simulink model "GreenCraneV1_mrhAdjust"  (R2025b)
settings: Solver=VariableStepAuto  StartTime=0.0  StopTime=40  RelTol=1e-3
model workspace (MATLAB code in the model file):
  | clear;
  | %% Hydraulics
  | 
  | %Liquid
  | rho = 875;
  | beta = 1000; %MPa
  | 
  | %Pump
  | pP = 6e6; %60 bar in pa
  | 
  | %Directional control valve
  | dp0 = 7e5; %Nominal pressure drop, Pa (stod 70e5)
  | Q0 = 10/6e4; %Nominal flow, m^3/s
  | Cd = 0.75; %Discharge coefficient
  | AdMax_SI = Q0/(Cd*(2/rho*dp0)^0.5); %Discharge area m^2
  | AdMax = AdMax_SI*1e6;
  | 
  | %cylinders (dummy)
  | d = 80; %mm
  | dr = 50; %mm
  | A = pi*d^2/4;
  | Ar = pi*dr^2/4;
  | Aa = A - Ar;
  | L0 = 1600; %mm
  | 
  | %Weight (bruker ikke lenger?)
  | m = 75*4 + 20 + 90; %kg
  | g = 9.81; %m/s^2
  | MG = m*g; %Force from weight
  | %inital postition
  | x_Init = 200; %mm
  | 
  | %% Geometric properties
  | 
  | % Cylinder Translation
  | Cx = 427; %mm translation from global coordinate
  | Cz = -1057; %mm translation
  | 
  | % Crane arm
  | theta_Init = 73.04- 90; %deg når kran er nede
  | thetaDot_Init = 0;
  | L1 = 3680; %mm length of beam
  | B1 = 100; %mm width of beam
  | H1 = 150; %mm height
  | t1 = 6; %mm thickness
  | revBasePinDia = 60; %mm of the pin in the main hinge
  | revBasePinLength = 185.5; %mm of the pin in the main hinge
  | 
  | %Cylinder
  | rEar = 35; %mm radius of the bearing ear
  | tEar = 30; %mm thickness of ear
  | earToCylTop = 52.45; %mm center of ear to top of cylinder in bottom pos
  | earToCylBot = 40.62; %mm center of ear to bottom cylinder in bottom pos
  | cylDia = 75; %mm Diameter of cylinger housing
  | cylLength = 682; %mm length of housing
  | rodLength = 565.26; %mm length of rod
  | rodDia = 35; %mm rod diameter
  | rodToCyl = 132; %mm Length in bottom pos from bottom of cylinder to bottom of rod without rod plate
  | revCylPinDia = 25; %mm diameter of the pin that the bearing of the top and bottom of cylinder revolves around
  | revCylPinLength = 84; %mm length of the pin
  | rPiston = 65/2; %mm radius of piston
  | tPiston = 40; %mm thickness of piston
  | 
  | %Ear top
  | abx = 564.99; %mm; in the bottom pos
  | aby = 133; %mm in the bottom pos
  | 
  | % PayLoad
  | L2 = 210; %mm of the whole weight block
  | B2 = 700; %mm
  | H2 = 300; %mm
  | dY_PL_Beam = 75; %mm center of beam to center of payload
  | 
  | %% Mass properties (mass and center of mass)
  | beam_mass = 410.675; %kg mass of payload and beam
  | beam_COM = [3043.56 63.40 0]; %mm
  | 
  | 
  | %% Inertia properties (Moments of inertia and products of inertia)
  | beam_MOI = [0.017432114  0.421942031  0.410722495];   % kg·m^2 Mulig feil rekkefølge
  | beam_POI = [0.011754324  -2.50964e-6  -5.072e-8];  % kg·m^2
  | %tro disse er i feil rekkefølge siden simscape bruker et annet aksesystem
undefined symbols (not defined in the file): X, Y, Z
libraries: sm_lib x37, fl_lib x16, nesl_utility x10, SimscapeFluids_lib x3
(part 2 of 2)

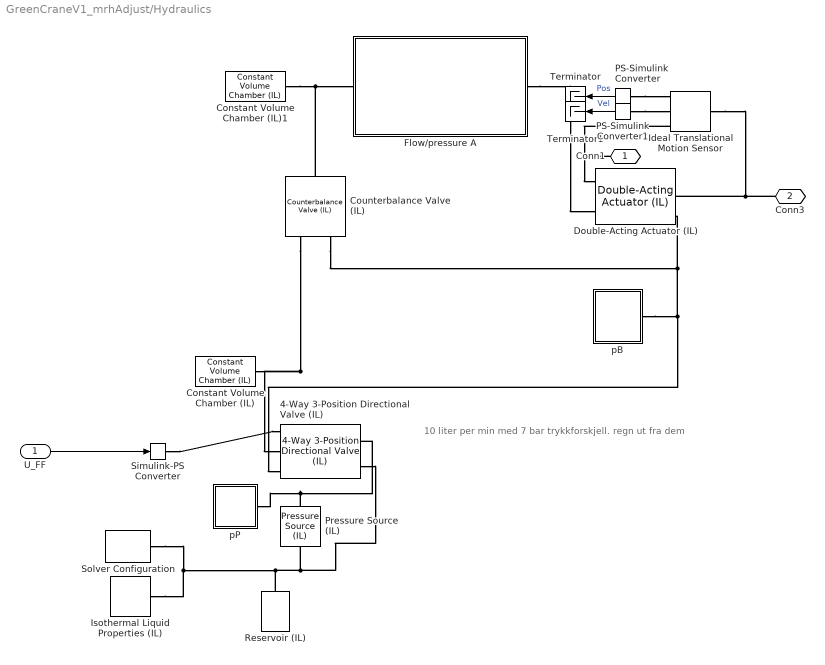
== system GreenCraneV1_mrhAdjust/Hydraulics ==
  note: 10 liter per min med 7 bar trykkforskjell. regn ut fra dem
  U_FF : Inport
  4-Way 3-Position Directional Valve (IL) : SimscapeFluids_lib/Isothermal Liquid/Valves & Orifices/Directional Control Valves/4-Way 3-Position Directional Valve (IL)  open_orifices_pos=fluids.isothermal_liquid.valves_orifices.directional_control_valves.enum.directional_valve_open_orifices_pos_neg.PA_BT  open_orifices_neu=fluids.isothermal_liquid.valves_orifices.directional_control_valves.enum.directional_valve_open_orifices_neutral.all_closed  open_orifices_neg=fluids.isothermal_liquid.valves_orifices.directional_control_valves.enum.directional_valve_open_orifices_pos_neg.PB_AT  neutral_assert_action=simscape.enum.assert.action.warn  area_spec=fluids.isothermal_liquid.valves_orifices.directional_control_valves.enum.directional_valve_area_spec.identical  valve_spec=fluids.isothermal_liquid.valves_orifices.directional_control_valves.enum.directional_valve_spec.linear  del_S_max=1 m  area_max=AdMax mm^2  del_S_TLU=[0, .00125, .0025, .00375, .005] m  valve_area_TLU=[1e-10, 1e-05, 4e-05, 6e-05, .0001] m^2  del_S_vol_flow_TLU=[0, .00125, .0025, .00375, .005] m  p_diff_TLU=[-.1, .3, .5, .7] MPa  vol_flow_TLU=[-1e-08, 2.2e-08, 2.8e-08, 3.4e-08; -9e-06, .00015, .0002, .00024; -.00036, .00063, .00081, .00096; -.00054, .00094, .0012, .0014; -.00091, .0016, .002, .0024] m^3/s  p_diff_TLU_const=[-.1, .3, .5, .7] MPa  vol_flow_TLU_const=[-.0009, .0016, .002, .0024] m^3/s  area_const=1e-4 m^2  area_leak=1e-10 m^2  area=inf m^2  Cd=Cd  Re_c=150  smoothing_factor=0.01  pressure_recovery=false  S_max_PA=1 m  del_S_max_PA=0.005 m  area_max_PA=1e-4 m^2  del_S_TLU_PA=[0, .00125, .0025, .00375, .005] m  valve_area_TLU_PA=[1e-10, 1e-05, 4e-05, 6e-05, .0001] m^2  del_S_vol_flow_TLU_PA=[0, .00125, .0025, .00375, .005] m  p_diff_TLU_PA=[-.1, .3, .5, .7] MPa  vol_flow_TLU_PA=[-1e-08, 2.2e-08, 2.8e-08, 3.4e-08; -9e-06, .00015, .0002, .00024; -.00036, .00063, .00081, .00096; -.00054, .00094, .0012, .0014; -.00091, .0016, .002, .0024] m^3/s  area_const_PA=1e-4 m^2  p_diff_TLU_const_PA=[-.1, .3, .5, .7] MPa  vol_flow_TLU_const_PA=[-.0009, .0016, .002, .0024] m^3/s  S_max_PB=-1 m  del_S_max_PB=0.005 m  area_max_PB=1e-4 m^2  del_S_TLU_PB=[0, .00125, .0025, .00375, .005] m  valve_area_TLU_PB=[1e-10, 1e-05, 4e-05, 6e-05, .0001] m^2  del_S_vol_flow_TLU_PB=[0, .00125, .0025, .00375, .005] m  p_diff_TLU_PB=[-.1, .3, .5, .7] MPa  vol_flow_TLU_PB=[-1e-08, 2.2e-08, 2.8e-08, 3.4e-08; -9e-06, .00015, .0002, .00024; -.00036, .00063, .00081, .00096; -.00054, .00094, .0012, .0014; -.00091, .0016, .002, .0024] m^3/s  area_const_PB=1e-4 m^2  p_diff_TLU_const_PB=[-.1, .3, .5, .7] MPa  vol_flow_TLU_const_PB=[-.0009, .0016, .002, .0024] m^3/s  S_max_AB=7.5e-3 m  del_S_max_AB=0.005 m  area_max_AB=1e-4 m^2  del_S_TLU_AB=[0, .00125, .0025, .00375, .005] m  valve_area_TLU_AB=[1e-10, 1e-05, 4e-05, 6e-05, .0001] m^2  del_S_vol_flow_TLU_AB=[0, .00125, .0025, .00375, .005] m  p_diff_TLU_AB=[-.1, .3, .5, .7] MPa  vol_flow_TLU_AB=[-1e-08, 2.2e-08, 2.8e-08, 3.4e-08; -9e-06, .00015, .0002, .00024; -.00036, .00063, .00081, .00096; -.00054, .00094, .0012, .0014; -.00091, .0016, .002, .0024] m^3/s  area_const_AB=1e-4 m^2  p_diff_TLU_const_AB=[-.1, .3, .5, .7] MPa  vol_flow_TLU_const_AB=[-.0009, .0016, .002, .0024] m^3/s  S_max_AT=-1 m  del_S_max_AT=0.005 m  area_max_AT=1e-4 m^2  del_S_TLU_AT=[0, .00125, .0025, .00375, .005] m  valve_area_TLU_AT=[1e-10, 1e-05, 4e-05, 6e-05, .0001] m^2  del_S_vol_flow_TLU_AT=[0, .00125, .0025, .00375, .005] m  p_diff_TLU_AT=[-.1, .3, .5, .7] MPa  vol_flow_TLU_AT=[-1e-08, 2.2e-08, 2.8e-08, 3.4e-08; -9e-06, .00015, .0002, .00024; -.00036, .00063, .00081, .00096; -.00054, .00094, .0012, .0014; -.00091, .0016, .002, .0024] m^3/s  area_const_AT=1e-4 m^2  p_diff_TLU_const_AT=[-.1, .3, .5, .7] MPa  vol_flow_TLU_const_AT=[-.0009, .0016, .002, .0024] m^3/s  S_max_BT=1 m  del_S_max_BT=0.005 m  area_max_BT=1e-4 m^2  del_S_TLU_BT=[0, .00125, .0025, .00375, .005] m  valve_area_TLU_BT=[1e-10, 1e-05, 4e-05, 6e-05, .0001] m^2  del_S_vol_flow_TLU_BT=[0, .00125, .0025, .00375, .005] m  p_diff_TLU_BT=[-.1, .3, .5, .7] MPa  vol_flow_TLU_BT=[-1e-08, 2.2e-08, 2.8e-08, 3.4e-08; -9e-06, .00015, .0002, .00024; -.00036, .00063, .00081, .00096; -.00054, .00094, .0012, .0014; -.00091, .0016, .002, .0024] m^3/s  area_const_BT=1e-4 m^2  p_diff_TLU_const_BT=[-.1, .3, .5, .7] MPa  vol_flow_TLU_const_BT=[-.0009, .0016, .002, .0024] m^3/s  S_max_PT=0 m  del_S_max_PT=0.005 m  area_max_PT=1e-4 m^2  del_S_TLU_PT=[0, .00125, .0025, .00375, .005] m  valve_area_TLU_PT=[1e-10, 1e-05, 4e-05, 6e-05, .0001] m^2  del_S_vol_flow_TLU_PT=[0, .00125, .0025, .00375, .005] m  p_diff_TLU_PT=[-.1, .3, .5, .7] MPa  vol_flow_TLU_PT=[-1e-08, 2.2e-08, 2.8e-08, 3.4e-08; -9e-06, .00015, .0002, .00024; -.00036, .00063, .00081, .00096; -.00054, .00094, .0012, .0014; -.00091, .0016, .002, .0024] m^3/s
      settings: InternalSimscapePortConfiguration="{\"Bottom\":[{\"id\":\"P\",\"label\":\"P\",\"type\":\"foundation.isothermal_liquid.isothermal_liquid\"},{\"id\":\"T\",\"label\":\"T\",\"type\":\"foundation.isothermal_liquid.isothermal_liquid\"}],\"Left\":[{\"id\":\"S\",\"label\":\"S\",\"type\":\"input\"}],\"Right\":[],\"Top\":[{\"id\":\"A\",\"label\":\"A\",\"type\":\"foundation.isothermal_liquid.isothermal_liquid\"},{\"id\":\"B\",\"label\":\"B\",\"type\":\"foundation.isothermal_liquid.isothermal_liquid\"}]}"
  Constant Volume Chamber (IL) : fl_lib/Isothermal Liquid/Elements/Constant Volume Chamber (IL)  volume=1 l  p_I_specify=on  p_I_priority=High  p_I=pP Pa  p_I_nominal_specify=off  p_I_nominal_value=1  p_I_nominal_unit=MPa
      settings: InternalSimscapePortConfiguration="{\"Bottom\":[],\"Left\":[{\"id\":\"A\",\"label\":\"A\",\"type\":\"foundation.isothermal_liquid.isothermal_liquid\"}],\"Right\":[],\"Top\":[]}"
  Constant Volume Chamber (IL)1 : fl_lib/Isothermal Liquid/Elements/Constant Volume Chamber (IL)  volume=1 l  p_I_specify=on  p_I_priority=High  p_I=pP Pa  p_I_nominal_specify=off  p_I_nominal_value=1  p_I_nominal_unit=MPa
      settings: InternalSimscapePortConfiguration="{\"Bottom\":[],\"Left\":[{\"id\":\"A\",\"label\":\"A\",\"type\":\"foundation.isothermal_liquid.isothermal_liquid\"}],\"Right\":[],\"Top\":[]}"
  Counterbalance Valve (IL) : SimscapeFluids_lib/Isothermal Liquid/Valves & Orifices/Pressure Control Valves/Counterbalance Valve (IL)  opening_spec=fluids.isothermal_liquid.valves_orifices.enum.PressureOpeningSpec.Linear  p_set_diff=5 MPa  p_max_diff=6 MPa  area_max=1e-4 m^2  area_leak=1e-10 m^2  p_diff_TLU=5 : 0.2 : 6 MPa  valve_area_TLU=[1e-10, 2e-05, 4e-05, 6e-05, 8e-05, .0001] m^2  p_diff_TLU_ref=5 : 0.2 : 6 MPa  vol_flow_TLU_ref=[6.4e-09, .0013, .0027, .0041, .0055, .007] m^3/s  pilot_ratio=3  back_ratio=4  Cd=0.64  Re_c=150  smoothing_factor=0.01  opening_dynamics=false  tau=0.1 s  check_p_crack=0.01 MPa  check_p_max=0.1 MPa  check_area_max=1e-4 m^2  check_p_diff_TLU=[0.01 : 0.01 : 0.1] MPa  check_area_TLU=[1e-10, 1e-05, 2e-05, 3e-05, 4e-05, 5e-05, 6e-05, 7.5e-05, 8.5e-05, .0001] m^2  check_vol_flow_TLU=[.000358, .045, .11, .191, .284, .39, .505, .63, .764, .905] .* 1e-3 m^3/s
      settings: InternalSimscapePortConfiguration="{\"Bottom\":[],\"Left\":[{\"id\":\"L\",\"label\":\"L\",\"type\":\"foundation.isothermal_liquid.isothermal_liquid\"}],\"Right\":[{\"id\":\"P\",\"label\":\"P\",\"type\":\"foundation.isothermal_liquid.isothermal_liquid\"},{\"id\":\"B\",\"label\":\"B\",\"type\":\"foundation.isothermal_liquid.isothermal_liquid\"}],\"Top\":[]}"
  Double-Acting Actuator (IL) : SimscapeFluids_lib/Isothermal Liquid/Actuators/Double-Acting Actuator (IL)  single_fluid=true  mech_orientation=foundation.enum.MechOrientationTranslational.Positive  piston_area_A=A mm^2  piston_area_B=Aa mm^2  stroke=L0 mm  dead_volume_A=1e-5 m^3  dead_volume_B=1e-5 m^3  pressure_spec=foundation.enum.pressure_spec.atmospheric  environment_pressure=0.101325 MPa  hardstop_model=simscape.enum.hardstop.smooth  stiff_coeff=1e10 N/m  damping_coeff=150 N*s/m  transition=0.1 mm  coeff_rest=0.7  v_tol=0.001 m/s  f_tol=0.001 N  cushion_A_spec=false  area_plunger_A=1e-4 m^2  length_plunger_A=1e-3 m  area_cushion_orifice_A=1e-6 m^2  area_leak_plunger_A=1e-7 m^2  p_crack_differential_A=0.01 MPa  press_max_differential_A=0.1 MPa  check_valve_area_max_A=1e-4 m^2  check_valve_area_leak_A=1e-10 m^2  smoothing_factor_A=0.01  cushion_B_spec=false  area_plunger_B=1e-4 m^2  length_plunger_B=1e-3 m  area_cushion_orifice_B=1e-6 m^2  area_leak_plunger_B=1e-7 m^2  p_crack_differential_B=0.01 MPa  press_max_differential_B=0.1 MPa  check_valve_area_max_B=1e-4 m^2  check_valve_area_leak_B=1e-10 m^2  smoothing_factor_B=0.01  friction_spec=false  breakaway_Coulomb_ratio=1.2  breakaway_velocity=0.1 m/s  preload_force=20 N  Coulomb_coeff=1e-6 N/Pa  viscous_coeff=100 N*s/m  leakage_spec=false  clearance=1e-4 m  piston_length=0.01 m  displacement_spec=foundation.enum.DisplacementSpec.Calculate  x0=x_Init mm  dynamic_compressibility=true  p0_A=pP Pa  p0_B=pP Pa  p_nominal_A=0.101325 MPa  p_nominal_B=0.101325 MPa
      settings: InternalSimscapePortConfiguration="{\"Bottom\":[],\"Left\":[{\"id\":\"C\",\"label\":\"C\",\"type\":\"foundation.mechanical.translational.translational\"},{\"id\":\"A\",\"label\":\"A\",\"type\":\"foundation.isothermal_liquid.isothermal_liquid\"}],\"Right\":[{\"id\":\"p_out\",\"label\":\"p\",\"type\":\"output\"},{\"id\":\"R\",\"label\":\"R\",\"type\":\"foundation.mechanical.translational.translational\"},{\"id\":\"B\",\"label\":\"B\",\"type\":\"foundation.isothermal_liquid.isothermal_liquid\"}],\"Top\":[]}"
  Flow/pressure A : Subsystem
  Ideal Translational Motion Sensor : fl_lib/Mechanical/Mechanical Sensors/Ideal Translational Motion Sensor  reference=foundation.enum.MeasurementReference.difference  acceleration_port=false  velocity_port=true  position_port=true  offset=x_Init mm
  Isothermal Liquid Properties (IL) : fl_lib/Isothermal Liquid/Utilities/Isothermal Liquid Properties (IL)  rho_L_atm=rho kg/m^3  bulk_modulus_model=foundation.enum.bulk_modulus_model.const  beta_gain=6  beta_L_atm=beta MPa  nu_atm=1.0034e-6 m^2/s  p_atm=0.101325 MPa  p_min=1 Pa  properties_range_check=simscape.enum.assert.action.error  air_fraction=0.005  polytropic_index=1.0  rho_g_atm=1.225 kg/m^3  air_dissolution_model=false  p_crit=3 MPa
  PS-Simulink Converter : nesl_utility/PS-Simulink Converter  PhysicalDomain=network_engine_domain  SubClassName=ps_output  LeftPortType=input  RightPortType=output  PseudoPeriodic=off  Frequencies=[]  VectorFormat=inherit  Unit=inherit  AffineConversion=off
  PS-Simulink Converter1 : nesl_utility/PS-Simulink Converter  PhysicalDomain=network_engine_domain  SubClassName=ps_output  LeftPortType=input  RightPortType=output  PseudoPeriodic=off  Frequencies=[]  VectorFormat=inherit  Unit=inherit  AffineConversion=off
  Pressure Source (IL) : fl_lib/Isothermal Liquid/Sources/Pressure Source (IL)  source_type=foundation.enum.constant_controlled.constant  pressure_differential=pP Pa
      settings: InternalSimscapePortConfiguration="{\"Bottom\":[],\"Left\":[{\"id\":\"A\",\"label\":\"A\",\"type\":\"foundation.isothermal_liquid.isothermal_liquid\"}],\"Right\":[{\"id\":\"B\",\"label\":\"B\",\"type\":\"foundation.isothermal_liquid.isothermal_liquid\"}],\"Top\":[]}"
  Reservoir (IL) : fl_lib/Isothermal Liquid/Elements/Reservoir (IL)  reservoir_type=foundation.enum.constant_controlled.constant  pressure_spec=foundation.enum.pressure_spec.atmospheric  reservoir_pressure=0.101325 MPa
  Simulink-PS Converter : nesl_utility/Simulink-PS Converter  PhysicalDomain=network_engine_domain  SubClassName=ps_input  LeftPortType=input  RightPortType=output  PseudoPeriodic=off  Frequencies=[]  NoiseDistribution=none  NoiseParameters=[]  Unit=1  AffineConversion=off  FilteringAndDerivatives=filter  SimscapeFilterOrder=2  InputFilterTimeConstant=0.001  UdotUserProvided=0
  Solver Configuration : nesl_utility/Solver Configuration  PhysicalDomain=network_engine_domain  SubClassName=solver  LeftPortType=input  RightPortType=generic  Tones=[]  Harmonics=[]  SimulateNoise=off  Profile=off  UseLocalSampling=off  EnableSwitchedLinearOptims=on  FrequencyDomain=off  UseCCode=off  RelTol=0.001  AbsTol=0.001  MinStep=1e-09  ToWorkspace=off  RevertToSquareIcSolve=off  NumHomotopyIterations=100  PhasorMode=off  PhasorModeNumHarmonics=1  ConsistencySolver=NEWTON_XTOL_AFTER_FTOL  IndexReductionMethod=DerivativeReplacement  DoDC=off  ResidualTolerance=1e-09  ConsistencyTolSource=GLOBAL  ConsistencyAbsTol=0.001  ConsistencyRelTol=0.001  ConsistencyTolFactor=0.001  UseLocalSolver=off  LocalSolverChoice=NE_BACKWARD_EULER_ADVANCER  ResolveIndetEquations=on  FunctionEvalNumThread=1  LocalSolverSampleTime=0.001  DoFixedCost=off  MaxNonlinIter=3  MaxModeIter=2  ComputeImpulses=off  ImpulseIterations=2  LinearAlgebra=auto  LinearAlgebraNumThread=0  EquationFormulation=NE_TIME_EF  DelaysMemoryBudget=1024  AutomaticFiltering=on  FilteringTimeConstant=0.001  PartitionStorageMethod=AS_NEEDED  PartitionMemoryBudget=1024  PartitionMethod=ROBUST  MultibodyUseLocalSolver=off  MultibodyLocalSolverChoice=ODE1  MultibodyLocalSolverSampleTime=0.001
  Terminator : Terminator
  Terminator1 : Terminator
  pB : Subsystem
  pP : Subsystem
  Conn1 : PMIOPort  Side=Right
  Conn3 : PMIOPort  Port=2  Side=Right
  wires:
  PS-Simulink Converter1/1 -> Terminator1/1  "Vel"
  PS-Simulink Converter/1 -> Terminator/1  "Pos"
  U_FF/1 -> Simulink-PS Converter/1
  connections:
  Counterbalance Valve (IL)/RConn1 -- pB/LConn1 -- 4-Way 3-Position Directional Valve (IL)/LConn3 -- Double-Acting Actuator (IL)/RConn3
  Pressure Source (IL)/RConn1 -- pP/LConn1 -- 4-Way 3-Position Directional Valve (IL)/RConn1
  Flow/pressure A/RConn1 -- Double-Acting Actuator (IL)/LConn2
  PS-Simulink Converter/LConn1 -- Ideal Translational Motion Sensor/RConn3
  Reservoir (IL)/LConn1 -- 4-Way 3-Position Directional Valve (IL)/RConn2 -- Pressure Source (IL)/LConn1 -- Solver Configuration/RConn1 -- Isothermal Liquid Properties (IL)/RConn1
  Ideal Translational Motion Sensor/LConn1 -- Conn3/RConn1 -- Double-Acting Actuator (IL)/RConn2
  PS-Simulink Converter1/LConn1 -- Ideal Translational Motion Sensor/RConn2
  Constant Volume Chamber (IL)/LConn1 -- Counterbalance Valve (IL)/RConn2 -- 4-Way 3-Position Directional Valve (IL)/LConn2
  Ideal Translational Motion Sensor/RConn1 -- Double-Acting Actuator (IL)/LConn1 -- Conn1/RConn1
  Counterbalance Valve (IL)/LConn1 -- Constant Volume Chamber (IL)1/LConn1 -- Flow/pressure A/LConn1
  Simulink-PS Converter/RConn1 -- 4-Way 3-Position Directional Valve (IL)/LConn1

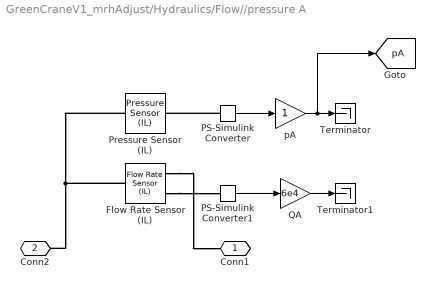
== system GreenCraneV1_mrhAdjust/Hydraulics/Flow//pressure A ==
  Flow Rate Sensor (IL) : fl_lib/Isothermal Liquid/Sensors/Flow Rate Sensor (IL)  sensor_type=foundation.enum.mass_volumetric_sensor.volumetric
      settings: InternalSimscapePortConfiguration="{\"Bottom\":[],\"Left\":[{\"id\":\"A\",\"label\":\"A\",\"type\":\"foundation.isothermal_liquid.isothermal_liquid\"}],\"Right\":[{\"id\":\"B\",\"label\":\"B\",\"type\":\"foundation.isothermal_liquid.isothermal_liquid\"},{\"id\":\"V\",\"label\":\"V\",\"type\":\"output\"}],\"Top\":[]}"
  PS-Simulink Converter : nesl_utility/PS-Simulink Converter  PhysicalDomain=network_engine_domain  SubClassName=ps_output  LeftPortType=input  RightPortType=output  PseudoPeriodic=off  Frequencies=[]  VectorFormat=inherit  Unit=inherit  AffineConversion=off
  PS-Simulink Converter1 : nesl_utility/PS-Simulink Converter  PhysicalDomain=network_engine_domain  SubClassName=ps_output  LeftPortType=input  RightPortType=output  PseudoPeriodic=off  Frequencies=[]  VectorFormat=inherit  Unit=inherit  AffineConversion=off
  Pressure Sensor (IL) : fl_lib/Isothermal Liquid/Sensors/Pressure Sensor (IL)  pressure_measure=foundation.enum.pressure_measure.gauge
      settings: InternalSimscapePortConfiguration="{\"Bottom\":[],\"Left\":[{\"id\":\"A\",\"label\":\"A\",\"type\":\"foundation.isothermal_liquid.isothermal_liquid\"}],\"Right\":[{\"id\":\"Pg\",\"label\":\"Pg\",\"type\":\"output\"}],\"Top\":[]}"
  QA : Gain  Gain=6e4
  Terminator : Terminator
  Terminator1 : Terminator
  pA : Gain
  Conn1 : PMIOPort  Side=Right
  Conn2 : PMIOPort  Port=2  Side=Left
  tag scope: pA=global
  wires:
  QA/1 -> Terminator1/1
  pA/1 -> [pA], Terminator/1
  PS-Simulink Converter/1 -> pA/1
  PS-Simulink Converter1/1 -> QA/1
  connections:
  Flow Rate Sensor (IL)/RConn2 -- PS-Simulink Converter1/LConn1
  Flow Rate Sensor (IL)/LConn1 -- Conn2/RConn1 -- Pressure Sensor (IL)/LConn1
  PS-Simulink Converter/LConn1 -- Pressure Sensor (IL)/RConn1
  Flow Rate Sensor (IL)/RConn1 -- Conn1/RConn1

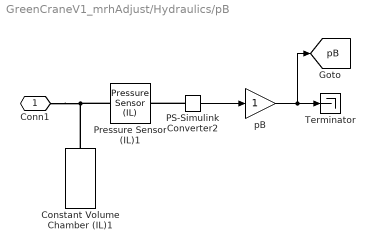
== system GreenCraneV1_mrhAdjust/Hydraulics/pB ==
  Constant Volume Chamber (IL)1 : fl_lib/Isothermal Liquid/Elements/Constant Volume Chamber (IL)  volume=1 l  p_I_specify=on  p_I_priority=High  p_I=20 bar  p_I_nominal_specify=off  p_I_nominal_value=1  p_I_nominal_unit=MPa
      settings: InternalSimscapePortConfiguration="{\"Bottom\":[],\"Left\":[{\"id\":\"A\",\"label\":\"A\",\"type\":\"foundation.isothermal_liquid.isothermal_liquid\"}],\"Right\":[],\"Top\":[]}"
  PS-Simulink Converter2 : nesl_utility/PS-Simulink Converter  PhysicalDomain=network_engine_domain  SubClassName=ps_output  LeftPortType=input  RightPortType=output  PseudoPeriodic=off  Frequencies=[]  VectorFormat=inherit  Unit=inherit  AffineConversion=off
  Pressure Sensor (IL)1 : fl_lib/Isothermal Liquid/Sensors/Pressure Sensor (IL)  pressure_measure=foundation.enum.pressure_measure.gauge
      settings: InternalSimscapePortConfiguration="{\"Bottom\":[],\"Left\":[{\"id\":\"A\",\"label\":\"A\",\"type\":\"foundation.isothermal_liquid.isothermal_liquid\"}],\"Right\":[{\"id\":\"Pg\",\"label\":\"Pg\",\"type\":\"output\"}],\"Top\":[]}"
  Terminator : Terminator
  pB : Gain
  Conn1 : PMIOPort  Side=Left
  tag scope: pB=global
  wires:
  PS-Simulink Converter2/1 -> pB/1
  pB/1 -> [pB], Terminator/1
  connections:
  PS-Simulink Converter2/LConn1 -- Pressure Sensor (IL)1/RConn1
  Conn1/RConn1 -- Pressure Sensor (IL)1/LConn1 -- Constant Volume Chamber (IL)1/LConn1

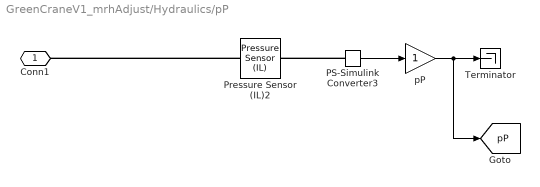
== system GreenCraneV1_mrhAdjust/Hydraulics/pP ==
  PS-Simulink Converter3 : nesl_utility/PS-Simulink Converter  PhysicalDomain=network_engine_domain  SubClassName=ps_output  LeftPortType=input  RightPortType=output  PseudoPeriodic=off  Frequencies=[]  VectorFormat=inherit  Unit=inherit  AffineConversion=off
  Pressure Sensor (IL)2 : fl_lib/Isothermal Liquid/Sensors/Pressure Sensor (IL)  pressure_measure=foundation.enum.pressure_measure.gauge
      settings: InternalSimscapePortConfiguration="{\"Bottom\":[],\"Left\":[{\"id\":\"A\",\"label\":\"A\",\"type\":\"foundation.isothermal_liquid.isothermal_liquid\"}],\"Right\":[{\"id\":\"Pg\",\"label\":\"Pg\",\"type\":\"output\"}],\"Top\":[]}"
  Terminator : Terminator
  pP : Gain
  Conn1 : PMIOPort  Side=Left
  tag scope: pP=global
  wires:
  PS-Simulink Converter3/1 -> pP/1
  pP/1 -> [pP], Terminator/1
  connections:
  PS-Simulink Converter3/LConn1 -- Pressure Sensor (IL)2/RConn1
  Pressure Sensor (IL)2/LConn1 -- Conn1/RConn1

== matlab function GreenCraneV1_mrhAdjust/Sinus ramp ==
  data: t input; u output
function u = valve_control(t)

t_ramp = 1;
t_hold = 4;
u_max  = 0.8;

if t < t_ramp
    % Smooth ramp up
    tau = t / t_ramp;
    u = u_max * 0.5 * (1 - cos(pi*tau));

elseif t < t_ramp + t_hold
    u = u_max;

elseif t < 2*t_ramp + t_hold
    % Smooth ramp to zero
    tau = (t - t_ramp - t_hold) / t_ramp;
    u = u_max * 0.5 * (1 + cos(pi*tau));

elseif t < 2*t_ramp + 2*t_hold
    u = 0;

elseif t < 3*t_ramp + 2*t_hold
    % Smooth ramp down
    tau = (t - 2*t_ramp - 2*t_hold) / t_ramp;
    u = -u_max * 0.5 * (1 - cos(pi*tau));

elseif t < 3*t_ramp + 3*t_hold
    u = -u_max;

else
    u = 0;
end

== matlab function GreenCraneV1_mrhAdjust/Feed forward/MATLAB Function ==
  data: t input; x output; x_dot output
function [x,x_dot] = fcn(t) 
a_max = 0.1; %Amplitude
f = 0.05; %frequency
x0 = 0.1; %offset

x = x0 - a_max*cos(2*pi*f*t); 
x_dot = a_max*2*pi*f*sin(2*pi*f*t);

== matlab function GreenCraneV1_mrhAdjust/Feed forward/MATLAB Function1 ==
  data: pA input; u_FF output; dP output; Q_req output; pB input; pP input; x_dot input; A parameter; Ar parameter; Q0 parameter
function [u_FF, dP, Q_req] = valveFeedForward(pA, pB, pP, x_dot, A, Ar, Q0)

% ---- Reference valve data ----
dp_ref = 7e5;      % reference pressure drop [Pa] er dette dp0?
Q0_ext = Q0;       % nominal valve flow at dp_ref (extend) [m^3/s]
Q0_ret = Q0;       % nominal valve flow at dp_ref (retract) [m^3/s]

dP_min = 1e5;            % numerical protection

% Convert cylinder areas from mm^2 to m^2
A  = A  * 1e-6;
Ar = Ar * 1e-6;

if x_dot > 0
    % Extension
    Q_req = A * x_dot;
    dP = pP - pA;
    Q0 = Q0_ext;
    dir = +1;

elseif x_dot < 0
    % Retraction
    Q_req = Ar * abs(x_dot);
    dP = pP - pB;
    Q0 = Q0_ret;
    dir = -1;

else
    u_FF = 0;
    dP = 0;
    Q_req = 0;
    return
end

% ---- Protect pressure ----
dP = max(dP, dP_min);

% ---- Pressure-compensated feed-forward ----
u_mag = (Q_req / Q0) * sqrt(dp_ref / dP);

% ---- Restore direction ----
u_FF = dir * u_mag;

% ---- Saturate ----
u_FF = max(min(u_FF, 1), -1);

end
